simulink model "Nonlinear_Backstepping_Controller_Design_Dr_CAN_03242018"  (R2014b)
settings: Solver=ode45  StartTime=0.0  StopTime=50  FixedStep=0.1  RelTol=1e-3
libraries: simulink x1
settings Model: CovSFcnEnable=on  Creator=tianwew  LastModifiedBy=zhoujie
settings OptimizationCC: UseDivisionForNetSlopeComputation=off  SimCompilerOptimization=off
settings DebuggingCC: SolverPrmCheckMsg=none  FrameProcessingCompatibilityMsg=error
settings RTWCC: RTWCompilerOptimization=off

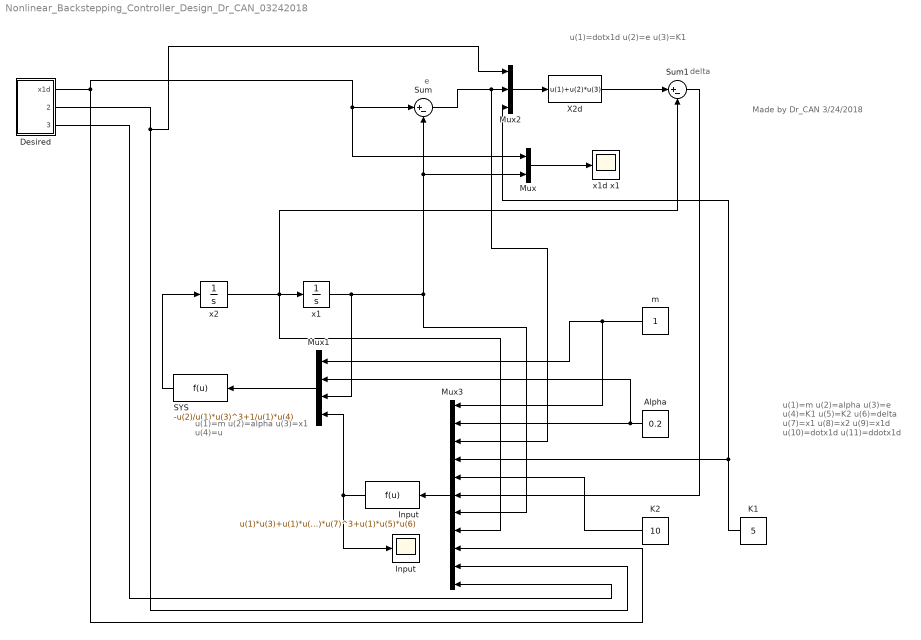
== system Nonlinear_Backstepping_Controller_Design_Dr_CAN_03242018 ==
  note: Made by Dr_CAN
      | 3/24/2018
  note: e
  note: u(1)=dotx1d
      | u(2)=e
      | u(3)=K1
  note: u(1)=m
      | u(2)=alpha
      | u(3)=x1
      | u(4)=u
  note: u(1)=m
      | u(2)=alpha
      | u(3)=e
      | u(4)=K1
      | u(5)=K2
      | u(6)=delta
      | u(7)=x1
      | u(8)=x2
      | u(9)=x1d
      | u(10)=dotx1d
      | u(11)=ddotx1d
  note: delta
  Alpha : Constant  Value=0.2
  Desired : Subsystem
  Input : Fcn  Expr=u(1)*u(3)+u(1)*u(11)+u(1)*u(4)*(u(10)-u(8))+u(2)*u(7)^3+u(1)*u(5)*u(6)
  "Input " : Scope
  K1 : Constant  Value=5
  K2 : Constant  Value=10
  Mux : Mux  Inputs=2
  Mux1 : Mux
  Mux2 : Mux  Inputs=3
  Mux3 : Mux  Inputs=11
  SYS : Fcn  Expr=-u(2)/u(1)*u(3)^3+1/u(1)*u(4)
  Sum : Sum  Inputs=|+-
  Sum1 : Sum  Inputs=|+-
  X2d : Fcn  Expr=u(1)+u(2)*u(3)
  m : Constant
  x1 : Integrator
  x1d x1 : Scope
  x2 : Integrator  UpperSaturationLimit=10  ZeroCross=off
  wires:
  x2/1 -> Sum1/2, x1/1, Mux3/8
  x1/1 -> Mux1/3, Mux/2, Sum/2, Mux3/7
  Mux/1 -> x1d x1/1
  Mux1/1 -> SYS/1
  SYS/1 -> x2/1
  Alpha/1 -> Mux1/2, Mux3/2
  m/1 -> Mux1/1, Mux3/1
  Desired/2(dotx1d) -> Mux3/10, Mux2/1
  Sum/1 -> Mux3/3, Mux2/2
  Mux2/1 -> X2d/1
  K1/1 -> Mux2/3, Mux3/4
  X2d/1 -> Sum1/1
  Mux3/1 -> Input/1
  K2/1 -> Mux3/5
  Sum1/1 -> Mux3/6
  Desired/3(ddotx1d) -> Mux3/11
  Desired/1(x1d) -> Mux3/9, Mux/1, Sum/1
  Input/1 -> "Input "/1, Mux1/4

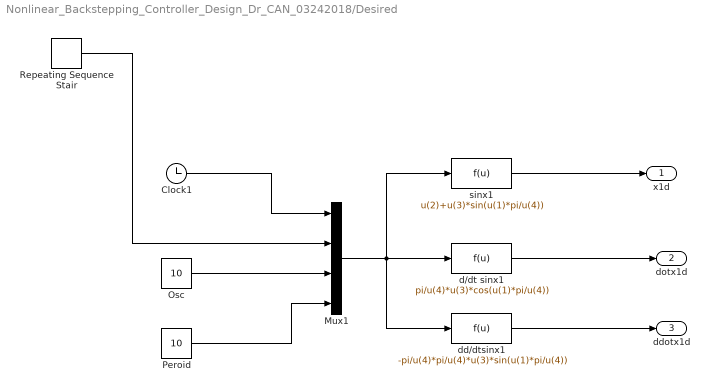
== system Nonlinear_Backstepping_Controller_Design_Dr_CAN_03242018/Desired ==
  Clock1 : Clock
      settings: Decimation=100
  Mux1 : Mux
  Osc : Constant  Value=10
  Peroid : Constant  Value=10
  Repeating Sequence Stair : simulink/Sources/Repeating Sequence Stair  OutValues=[3 10 1 0 4].'  tsamp=10  OutMin=[]  OutMax=[]  OutDataTypeStr=double  OutputDataTypeScalingMode=double  OutDataType=fixdt(0,8)  ConRadixGroup=Best Precision: Vector-wise  OutScaling=2^-12
  d/dt sinx1 : Fcn  Expr=pi/u(4)*u(3)*cos(u(1)*pi/u(4))
  dd/dtsinx1 : Fcn  Expr=-pi/u(4)*pi/u(4)*u(3)*sin(u(1)*pi/u(4))
  sinx1 : Fcn  Expr=u(2)+u(3)*sin(u(1)*pi/u(4))
  x1d : Outport
  dotx1d : Outport  Port=2
  ddotx1d : Outport  Port=3
  wires:
  Repeating Sequence Stair/1 -> Mux1/2
  Clock1/1 -> Mux1/1
  Mux1/1 -> sinx1/1, dd/dtsinx1/1, d/dt sinx1/1
  Osc/1 -> Mux1/3
  Peroid/1 -> Mux1/4
  d/dt sinx1/1 -> dotx1d/1
  dd/dtsinx1/1 -> ddotx1d/1
  sinx1/1 -> x1d/1
